simulink model "BBModel_Run"  (R2024a)
settings: Solver=ode4  StartTime=0.2  StopTime=1  FixedStep=1e-8  RelTol=1e-3
values from neighbouring files (symbols this model uses):
  alpha = 0.05    [parameter.m]
  Cdin = 0    [parameter.m]
  Cdout = 0    [parameter.m]
  D2 = 54.06e-3    (= 0.05406)    [parameter.m]
  D_ball = (D2 - d1) / 2    (= 0.00685)    [parameter.m]
  F = 200    [parameter.m]
  g = 9.81    [parameter.m]
  Nb = 9    [parameter.m]
  Ts = 1e-7    (= 1e-07)    [parameter.m]
  u0 = zeros(ndof,1)    [parameter.m]
  v0 = zeros(ndof,1)    [parameter.m]
  ws = 2 * pi * fs    (= 314.159265359)    [parameter.m]
undefined symbols (not defined in the file or in its folder): param
settings Model: Creator=elboun1  LastModifiedBy=nadaelbou
settings ModelReferenceCC: EnableRefExpFcnMdlSchedulingChecks=on
settings RTWCC: GPUComputeCapability=3.5

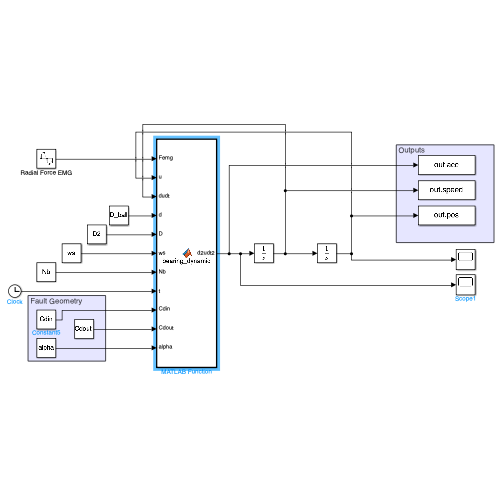
[thumbnail: Simulink's stored preview of the top-level diagram]
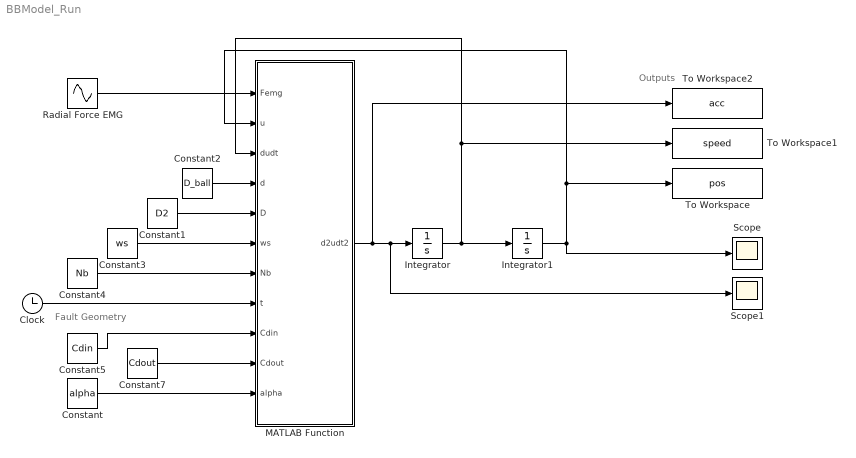
== system BBModel_Run ==
  note: Outputs
  note: Fault Geometry
  Clock : Clock
  Constant : Constant  Value=alpha
  Constant1 : Constant  Value=D2
  Constant2 : Constant  Value=D_ball
  Constant3 : Constant  Value=ws
  Constant4 : Constant  Value=Nb
  Constant5 : Constant  Value=Cdin
  Constant7 : Constant  Value=Cdout
  Integrator : Integrator  InitialCondition=v0
  Integrator1 : Integrator  InitialCondition=u0
  MATLAB Function : MATLAB Function  TreatAsAtomicUnit=on
  Radial Force EMG : Sin  Amplitude=F  Frequency=ws  SampleTime=Ts
  Scope : Scope
  Scope1 : Scope
  To Workspace : ToWorkspace  VariableName=pos  SaveFormat=Timeseries  SampleTime=-1
  To Workspace1 : ToWorkspace  VariableName=speed  SaveFormat=Timeseries  SampleTime=-1
  To Workspace2 : ToWorkspace  VariableName=acc  SaveFormat=Timeseries  SampleTime=-1
  wires:
  Integrator/1 -> To Workspace1/1, MATLAB Function/3(dudt), Integrator1/1
  Integrator1/1 -> To Workspace/1, MATLAB Function/2(u), Scope/1
  MATLAB Function/1(d2udt2) -> To Workspace2/1, Integrator/1, Scope1/1
  Constant3/1 -> MATLAB Function/6(ws)
  Constant1/1 -> MATLAB Function/5(D)
  Constant2/1 -> MATLAB Function/4(d)
  Constant4/1 -> MATLAB Function/7(Nb)
  Clock/1 -> MATLAB Function/8(t)
  Radial Force EMG/1 -> MATLAB Function/1(Femg)
  Constant5/1 -> MATLAB Function/9(Cdin)
  Constant7/1 -> MATLAB Function/10(Cdout)
  Constant/1 -> MATLAB Function/11(alpha)

== matlab function BBModel_Run/MATLAB Function ==
  data: Femg input; u input; dudt input; d2udt2 output; param parameter; g parameter; d input; D input; ws input; Nb input; t input; Cdin input; Cdout input; alpha input
function d2udt2 = bearing_dynamic(Femg, u, dudt, param, g, d, D, ws, Nb, t, Cdin, Cdout, alpha)

    % Inverse mass matrix
    Minv = diag(1 ./ param.m);
    
    % Calculate angular position of the second ball
    wc = ws / 2 * (1 - d / D);
    theta0 = 0.01;  % Initial angle for second ball
    theta = mod(2 * pi * (2 - 1) / Nb + wc * t + theta0, 2 * pi);
    
    % Determine displacements and velocities based on angular position
    if (theta > 270 * pi / 180) && (theta > 270 * pi / 180 + alpha)
        Xi = u(3) - u(2) + Cdin;
        Vi = dudt(3) - dudt(2);
        Xo = u(4) - u(3) + Cdout;
        Vo = dudt(4) - dudt(3);
    else 
        Xi = u(3) - u(2);
        Vi = dudt(3) - dudt(2);
        Xo = u(4) - u(3);
        Vo = dudt(4) - dudt(3);
    end 
    
    % Compute damping coefficients
    if Vo == 0 || Vi == 0 
        ch_i = param.c(1);
        ch_o = param.c(2);
    else 
        r = 0.6;
        eps = 9 * sqrt(5) * (1 - r^2) / (10 * r^2);
        ch_i = eps * Xi^3 / 2;
        ch_o = eps * Xo^3 / 2; 
    end 
    
    % Damping matrix
    C = [0, 0, 0, 0;
         0, ch_i, -ch_i, 0;
         0, -ch_i, ch_i + ch_o, -ch_o;
         0, 0, -ch_o, ch_o];
    
    % Stiffness matrix
    K = [param.k(1), -param.k(1), 0, 0;
         -param.k(1), param.k(1) + param.k(2), -param.k(2), 0;
         0, -param.k(2), param.k(2) + param.k(3), -param.k(3);
         0, 0, -param.k(3), param.k(3) + param.k(4)];
    
    % Hertzian contact forces
    Fhi = param.khertz(1) * sign(Xi) * abs(Xi)^(3/2);
    Fho = param.khertz(2) * sign(Xo) * abs(Xo)^(3/2);
    
    % Force calculation considering weight rotor
    if (theta > pi * 5 / 4) && (theta <= pi * 7 / 4)
        F = [Femg * cos(wc * t); zeros(3,1)] ...
            - param.m * g * sin(wc - ws) ...
            + [0; Fhi; Fho - Fhi; -Fho] ...
            - (param.shaft * ones(4,1) * g * sin(mod(theta, pi / 2)));
    else 
        F = [Femg * cos(wc * t); zeros(3,1)] ...
            - param.m * g * sin(wc - ws) ...
            + [0; Fhi; Fho - Fhi; -Fho];
    end 
    
    % Compute acceleration
    d2udt2 = Minv * (F - C * dudt - K * u);
    
end
